simulink model "Kubon_lab10_2_sim"  (R2020b)
settings: Solver=VariableStepAuto  StartTime=0.0  StopTime=T_stop  RelTol=1e-3
values from neighbouring files (symbols this model uses):
  dTkz = 2.0    (= 2)    [Kubon_lab10.m]    (also in Kubon_lab9.m = 0)
  dTzew = 0.0    (= 0)    [Kubon_lab10.m]    (also in Kubon_lab9.m)
  L1 = [(Cv2*a_1) (a_1*(ks2+a_1+k0))]    [Kubon_lab10.m]    (also in Kubon_lab8.m = M2_)
  L2 = [(Cv2*ks1) ((k0*ks2)+(ks1*(a_1+ks2+k0)))]    [Kubon_lab10.m]    (also in Kubon_lab8.m = [ a1 ])
  L3 = (k0*a_1+a_1*a_1)    (= 1108800)    [Kubon_lab10.m]    (also in Kubon_lab8.m = [ a1 ])
  L4 = [(Cv1+ks2) (k0*ks1+(a_1*ks1)+(ks2*(a_1+ks1+k0)))]    [Kubon_lab10.m]    (also in Kubon_lab8.m = M1_)
  M1 = [(Cv1*Cv2) (Cv1*a_1+Cv1*ks2+Cv1*k0+Cv2*a_1+Cv2*ks1+Cv2*k0) (a_1^2+a_1*ks2+a_1*k0  +a_1*ks1+ks1*ks2+ks1*k0    +k0*ks2)]    [Kubon_lab10.m]    (also in Kubon_lab8.m = [A1*A2 , A1*a1+A1*a2+A2*a1 , a1*a2])
  M2 = M1    [Kubon_lab10.m]    (also in Kubon_lab8.m)
  M3 = M2    [Kubon_lab10.m]    (also in Kubon_lab8.m)
  M4 = M3    [Kubon_lab10.m]    (also in Kubon_lab8.m)
  t0 = 50.0    (= 50)    [Kubon_lab10.m]    (also in Kubon_lab4.m = 5; Kubon_lab5.m = 0; Kubon_lab6.m = 5; Kubon_lab6_test.m = 0)
  Tw10 = ( (a_1*b_1*Tkz0)+ks1*(ks1+a_1+2*k0)*Tzew0 )/( (b_1^2)-(k0*(k0+a_1)) )    (= 9.848)    [Kubon_lab10.m]    (also in Kubon_lab9.m = 20)
  Tw20 = ( (k0+a_1)*Tw10+ks1*Tzew0 )/( k0+a_1+ks1 )    (= 5.256)    [Kubon_lab10.m]    (also in Kubon_lab9.m = 15)
settings Model: Creator=pkubo  LastModifiedBy=pkubo

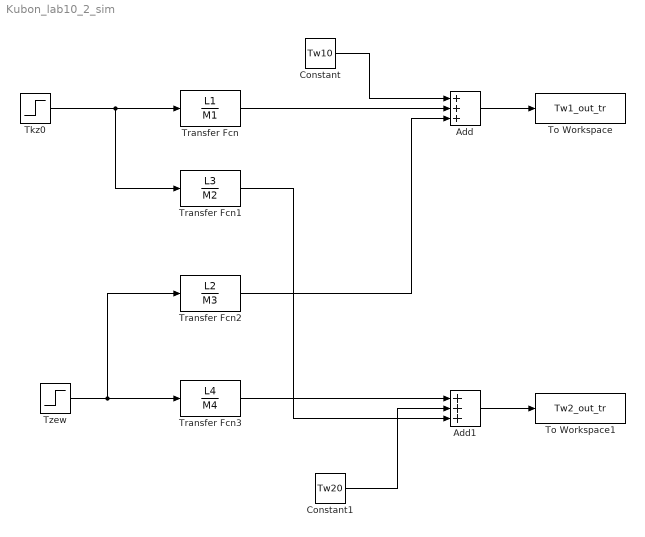
== system Kubon_lab10_2_sim ==
  Add : Sum  Inputs=+++
  Add1 : Sum  Inputs=+++
  Constant : Constant  Value=Tw10
  Constant1 : Constant  Value=Tw20
  Tkz0 : Step  Time=t0  After=dTkz  SampleTime=0
  To Workspace : ToWorkspace  VariableName=Tw1_out_tr  SampleTime=-1
  To Workspace1 : ToWorkspace  VariableName=Tw2_out_tr  SampleTime=-1
  Transfer Fcn : TransferFcn  Numerator=L1  Denominator=M1
  Transfer Fcn1 : TransferFcn  Numerator=L3  Denominator=M2
  Transfer Fcn2 : TransferFcn  Numerator=L2  Denominator=M3
  Transfer Fcn3 : TransferFcn  Numerator=L4  Denominator=M4
  Tzew : Step  Time=t0  After=dTzew  SampleTime=0
  wires:
  Tzew/1 -> Transfer Fcn2/1, Transfer Fcn3/1
  Tkz0/1 -> Transfer Fcn1/1, Transfer Fcn/1
  Transfer Fcn2/1 -> Add/3
  Transfer Fcn3/1 -> Add1/1
  Add1/1 -> To Workspace1/1
  Constant1/1 -> Add1/2
  Add/1 -> To Workspace/1
  Constant/1 -> Add/1
  Transfer Fcn/1 -> Add/2
  Transfer Fcn1/1 -> Add1/3
